simulink model "LectureVersion_Stage01_Heater"  (R2021b)
settings: Solver=VariableStepAuto  StartTime=0.0  StopTime=10.0  RelTol=1e-3
model workspace (MAT data in the model file):
  M_heater_air = 3600
  T_heater = 50
  c_air = 1005.4
  m_room_air = 1470
settings Model: Creator=jim  LastModifiedBy=jim

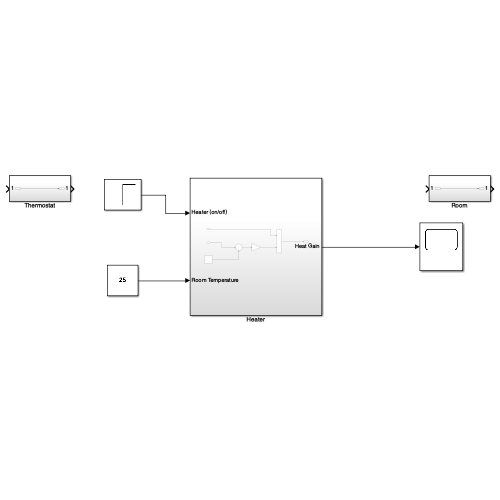
[thumbnail: Simulink's stored preview of the top-level diagram]
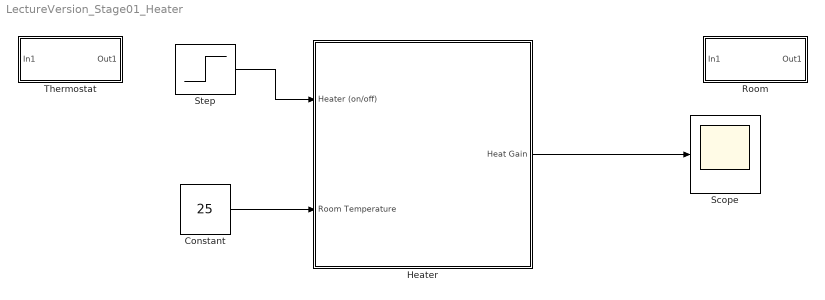
== system LectureVersion_Stage01_Heater ==
  Constant : Constant  Value=25
  Heater : Subsystem
  Room : Subsystem
  Scope : Scope
  Step : Step  Time=4  SampleTime=0
  Thermostat : Subsystem
  wires:
  Step/1 -> Heater/1(Heater (on/off))
  Constant/1 -> Heater/2(Room Temperature)
  Heater/1(Heat Gain) -> Scope/1

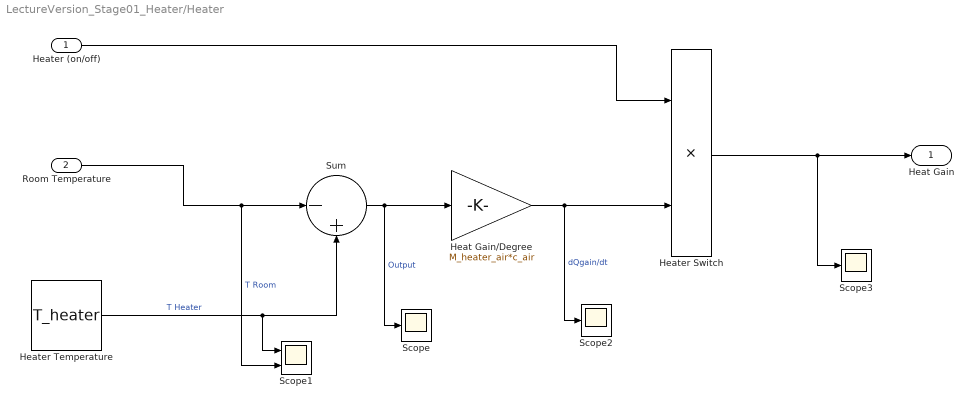
== system LectureVersion_Stage01_Heater/Heater ==
  Heater (on/off) : Inport
  Room Temperature : Inport  Port=2
  Heat Gain/Degree : Gain  Gain=M_heater_air*c_air
  Heater Switch : Product
  Heater Temperature : Constant  Value=T_heater
  Scope : Scope
  Scope1 : Scope  NumInputPorts=2
  Scope2 : Scope
  Scope3 : Scope
  Sum : Sum  Inputs=|-+
  Heat Gain : Outport
  wires:
  Sum/1 -> Scope/1, Heat Gain/Degree/1  "Output"
  Room Temperature/1 -> Scope1/2, Sum/1  "T Room"
  Heater Temperature/1 -> Scope1/1, Sum/2  "T Heater"
  Heater (on/off)/1 -> Heater Switch/1
  Heater Switch/1 -> Scope3/1, Heat Gain/1
  Heat Gain/Degree/1 -> Scope2/1, Heater Switch/2  "dQgain/dt"

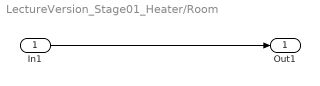
== system LectureVersion_Stage01_Heater/Room ==
  In1 : Inport
  Out1 : Outport
  wires:
  In1/1 -> Out1/1

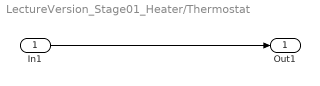
== system LectureVersion_Stage01_Heater/Thermostat ==
  In1 : Inport
  Out1 : Outport
  wires:
  In1/1 -> Out1/1
